simulink model "slbb"  (Simulink 2.20)
settings: Solver=ode5  StartTime=0.0  StopTime=1000  FixedStep=0.1  MaxStep=0.1  RelTol=1e-3  AbsTol=1e-6
PreLoadFcn:
  | initbb
CloseFcn:
  | AnimBbFigTitle = [winName, ': Ball & Beam Animation']; AnimBbFigH = findobj(0,'Name',AnimBbFigTitle); close(AnimBbFigH)
settings Model: SaveTime=off  SaveOutput=off  ConsistencyChecking=off  RTWPlaceOutputsASAP=off  RTWTemplateMakefile=grt_unix.tmf

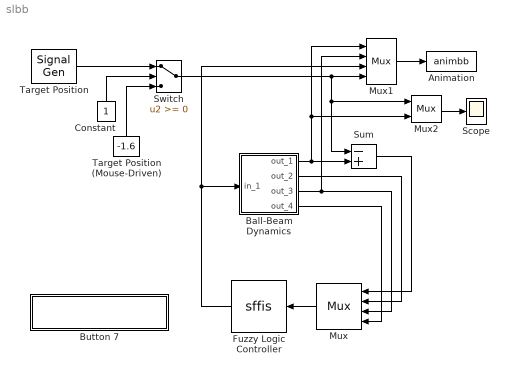
== system slbb ==
  Animation : S-Function  FunctionName=animbb  PortCounts=[]  SFunctionModules=''
  Ball-Beam Dynamics : Subsystem  mask(Ball-Beam Dynamics){@1=[0 0 0 0]}
      mask prompts: @1 "Initial Conditions:"
      mask help: Ball-Beam Dynamics
      mask init:
      | init_cond = @1;
      mask Help: Dynamics of the ball and beam system
      mask Display: plot(-4,-1,4,5,[0 -1 1 0 3 2.9 -3 -2.9 0],[2 0 0 2 3 3.1 1.1 1.0 2],0.3*cos(linspace(0,2*pi,9))+2,0.3*sin(linspace(0,2*pi,9))+3.1);
  Button 7 : Subsystem
      settings: OpenFcn=initbb
      mask Display: disp('Variable Initialization')
  Constant : Constant  Orientation=up  Value=1
  Fuzzy Logic Controller : S-Function  Orientation=left  FunctionName=sffis  Parameters=fismatrix  PortCounts=[]  SFunctionModules=sfsup  mask(FIS){@1=fismatrix}
      mask prompts: @1 "FIS Matrix:"
      mask help: FIS
      mask init:
      | fismatrix = @1;
      mask Help: Fuzzy Inference System
      mask Display: plot(0, -0.3, 6, -0.3, 0, 1.2, 6, 1.2, [0 6], [0 0], [1 2 3],[0 1 0],[2 3 4],[0 1 0],[3 4 5],[0 1 0])
  Mux : Mux  Orientation=left  Inputs=4
  Mux1 : Mux  Inputs=4
  Mux2 : Mux  Inputs=2
  Scope : Scope
      settings: TickLabels=on  TimeRange=10.000000  YMin=-2.000000  YMax=2.000000  SaveToWorkspace=off  SaveName=ScopeData
  Sum : Sum  Inputs=-+
  Switch : Switch  Threshold=0
  Target Position : SignalGenerator  WaveForm=square  Amplitude=1.600000  Frequency=0.500000  Units=rad/sec
  Target Position (Mouse-Driven) : Constant  Orientation=up  Value=-1.6
  wires:
  Mux2/1 -> Scope/1
  Switch/1 -> Mux2/1, Sum/1, Mux1/4
  Sum/1 -> Mux/1
  Ball-Beam Dynamics/2(out_2) -> Mux/2
  Ball-Beam Dynamics/3(out_3) -> Mux/3, Mux1/2
  Ball-Beam Dynamics/4(out_4) -> Mux/4
  Target Position (Mouse-Driven)/1 -> Switch/3
  Constant/1 -> Switch/2
  Target Position/1 -> Switch/1
  Ball-Beam Dynamics/1(out_1) -> Mux2/2, Mux1/1, Sum/2
  Mux/1 -> Fuzzy Logic Controller/1
  Mux1/1 -> Animation/1
  Fuzzy Logic Controller/1 -> Mux1/3, Ball-Beam Dynamics/1(in_1)

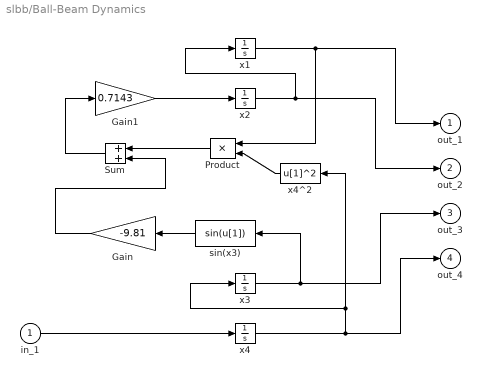
== system slbb/Ball-Beam Dynamics ==
  in_1 : Inport  Port=1  PortWidth=-1  SampleTime=-1
  Gain : Gain  Orientation=left  Gain=-9.81
  Gain1 : Gain  Gain=0.7143
  Product : Product  Orientation=left  Inputs=2
  Sum : Sum  Orientation=left  Inputs=++
  sin(x3) : Fcn  Orientation=left  Expr=sin(u[1])
  x1 : Integrator  ExternalReset=none  InitialConditionSource=internal  InitialCondition=init_cond(1)  LimitOutput=off  UpperSaturationLimit=inf  LowerSaturationLimit=-inf  ShowSaturationPort=off  ShowStatePort=off  AbsoluteTolerance=auto
  x2 : Integrator  ExternalReset=none  InitialConditionSource=internal  InitialCondition=init_cond(2)  LimitOutput=off  UpperSaturationLimit=inf  LowerSaturationLimit=-inf  ShowSaturationPort=off  ShowStatePort=off  AbsoluteTolerance=auto
  x3 : Integrator  ExternalReset=none  InitialConditionSource=internal  InitialCondition=init_cond(3)  LimitOutput=off  UpperSaturationLimit=inf  LowerSaturationLimit=-inf  ShowSaturationPort=off  ShowStatePort=off  AbsoluteTolerance=auto
  x4 : Integrator  ExternalReset=none  InitialConditionSource=internal  InitialCondition=init_cond(4)  LimitOutput=off  UpperSaturationLimit=inf  LowerSaturationLimit=-inf  ShowSaturationPort=off  ShowStatePort=off  AbsoluteTolerance=auto
  x4^2 : Fcn  Orientation=left  Expr=u[1]^2
  out_1 : Outport  Port=1  InitialOutput=0
  out_2 : Outport  Port=2  InitialOutput=0
  out_3 : Outport  Port=3  InitialOutput=0
  out_4 : Outport  Port=4  InitialOutput=0
  wires:
  in_1/1 -> x4/1
  x2/1 -> out_2/1, x1/1
  x1/1 -> Product/1, out_1/1
  x4^2/1 -> Product/2
  sin(x3)/1 -> Gain/1
  Product/1 -> Sum/1
  Gain/1 -> Sum/2
  Sum/1 -> Gain1/1
  Gain1/1 -> x2/1
  x4/1 -> x3/1, x4^2/1, out_4/1
  x3/1 -> sin(x3)/1, out_3/1

== system slbb/Button 7 ==
